simulink subsystem "PowerSplitDriveUnitBasic_refsub"  (R2020b)
settings: Solver=VariableStepAuto  StartTime=0.0  StopTime=10.0  RelTol=1e-3
libraries: nesl_utility x4, fl_lib x2
settings Model: Creator=isaacito  LastModifiedBy=isaacito

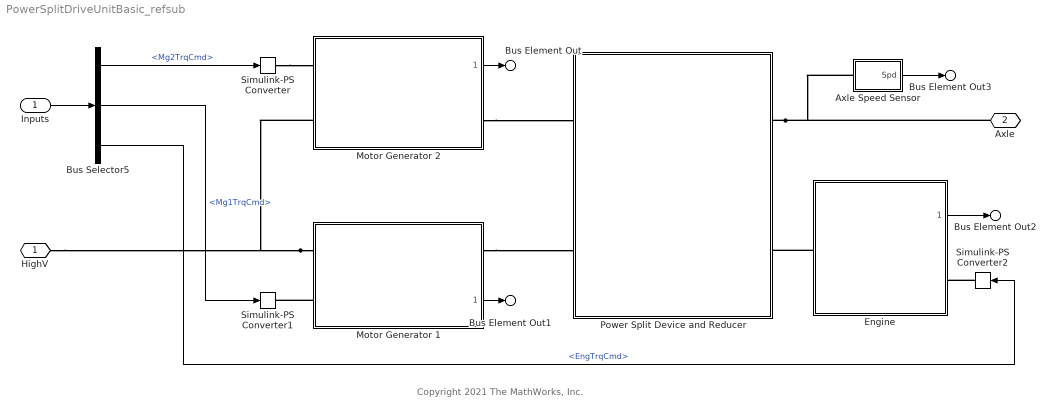
== system PowerSplitDriveUnitBasic_refsub ==
  note: Copyright 2021 The MathWorks, Inc.
  Inputs : Inport
  Axle Speed Sensor : Subsystem
  Bus Selector5 : BusSelector  OutputSignals=Mg2TrqCmd,Mg1TrqCmd,EngTrqCmd
  Engine : Subsystem  ReferencedSubsystem=EngineBasic_refsub
  Motor Generator 1 : Subsystem  ReferencedSubsystem=MotorGenerator1Basic_refsub
      settings: PortSchema="{\"entries\":[{\"content\":{\"sides\":[{\"content\":{\"connectorIds\":[\"LConn1\",\"LConn2\"]},\"type\":\"ConnectorPlacement.EquallySpacedRectSide\",\"uuid\":\"3f13e6b9-9785-470e-b4e7-2230544192d3\"},{\"content\":{\"connectorIds\":[\"RConn1\",\"Out1\"],\"side\":\"RIGHT\"},\"type\":\"ConnectorPlacement.EquallySpacedRectSide\",\"uuid\":\"c86dc6d1-f3ea-46c4-b113-258136dcfee4\"},{\"content\":{\"connectorIds\":[],\"side\":\"TOP\"},\"type\":\"ConnectorPlacement.EquallySpacedRectSide\",\"uuid\":\"633c827b-a9f1-4506-b379-ba2a2b41c3a4\"},{\"content\":{\"connectorIds\":[],\"side\":\"HIDDEN\"},\"type\":\"ConnectorPlacement.EquallySpacedRectSide\",\"uuid\":\"493696b9-c4b5-4599-b165-b63d9ea3db6c\"}]},\"type\":\"ConnectorPlacement.EquallySpacedConnector\",\"uuid\":\"29b0ca39-3f61-4a79-b1ec-51b22406ccf5\"}],\"packageUris\":[\"http://schema.mathworks.com/mf0/Connector/R2020b\"],\"version\":\"1.0\"}"
  Motor Generator 2 : Subsystem  ReferencedSubsystem=MotorGenerator2Basic_refsub
      settings: PortSchema="{\"entries\":[{\"content\":{\"sides\":[{\"content\":{\"connectorIds\":[\"LConn2\",\"LConn1\"]},\"type\":\"ConnectorPlacement.EquallySpacedRectSide\",\"uuid\":\"fb1ae627-2a11-4cdc-b40f-1f1ad643affe\"},{\"content\":{\"connectorIds\":[\"Out1\",\"RConn1\"],\"side\":\"RIGHT\"},\"type\":\"ConnectorPlacement.EquallySpacedRectSide\",\"uuid\":\"00f90b97-65a5-4f07-9d46-c4d934bbcebd\"},{\"content\":{\"connectorIds\":[],\"side\":\"TOP\"},\"type\":\"ConnectorPlacement.EquallySpacedRectSide\",\"uuid\":\"1403ad56-fcb4-428e-96ec-7b36e4f507b4\"},{\"content\":{\"connectorIds\":[],\"side\":\"HIDDEN\"},\"type\":\"ConnectorPlacement.EquallySpacedRectSide\",\"uuid\":\"421b449c-9b3e-4f4b-a79f-ec7613821770\"}]},\"type\":\"ConnectorPlacement.EquallySpacedConnector\",\"uuid\":\"1887aacf-d3d5-4d1b-946b-79f82bd43283\"}],\"packageUris\":[\"http://schema.mathworks.com/mf0/Connector/R2020b\"],\"version\":\"1.0\"}"
  Power Split Device and Reducer : Subsystem  ReferencedSubsystem=PowerSplitDeviceBasic_refsub
  Simulink-PS Converter : nesl_utility/Simulink-PS Converter  PhysicalDomain=network_engine_domain  SubClassName=ps_input  LeftPortType=input  RightPortType=output  PseudoPeriodic=off  Frequencies=[]  NoiseDistribution=none  NoiseParameters=[]  Unit=N*m  AffineConversion=off  FilteringAndDerivatives=provide  SimscapeFilterOrder=1  InputFilterTimeConstant=0.001  UdotUserProvided=0
  Simulink-PS Converter1 : nesl_utility/Simulink-PS Converter  PhysicalDomain=network_engine_domain  SubClassName=ps_input  LeftPortType=input  RightPortType=output  PseudoPeriodic=off  Frequencies=[]  NoiseDistribution=none  NoiseParameters=[]  Unit=N*m  AffineConversion=off  FilteringAndDerivatives=provide  SimscapeFilterOrder=1  InputFilterTimeConstant=0.001  UdotUserProvided=0
  Simulink-PS Converter2 : nesl_utility/Simulink-PS Converter  PhysicalDomain=network_engine_domain  SubClassName=ps_input  LeftPortType=input  RightPortType=output  PseudoPeriodic=off  Frequencies=[]  NoiseDistribution=none  NoiseParameters=[]  Unit=N*m  AffineConversion=off  FilteringAndDerivatives=provide  SimscapeFilterOrder=1  InputFilterTimeConstant=0.001  UdotUserProvided=0
  HighV : PMIOPort  Side=Left
  Axle : PMIOPort  Port=2  Side=Right
  Bus Element Out : Outport  PortName=Info  Element=mg2
  Bus Element Out1 : Outport  PortName=Info  Element=mg1
  Bus Element Out2 : Outport  PortName=Info  Element=eng
  Bus Element Out3 : Outport  PortName=Info  Element=AxleSpd
  wires:
  Motor Generator 2/1 -> Bus Element Out/1
  Motor Generator 1/1 -> Bus Element Out1/1
  Engine/1 -> Bus Element Out2/1
  Bus Selector5/3 -> Simulink-PS Converter2/1  "<EngTrqCmd>"
  Bus Selector5/2 -> Simulink-PS Converter1/1  "<Mg1TrqCmd>"
  Inputs/1 -> Bus Selector5/1
  Axle Speed Sensor/1(Spd) -> Bus Element Out3/1
  Bus Selector5/1 -> Simulink-PS Converter/1  "<Mg2TrqCmd>"
  connections:
  Motor Generator 1/LConn1 -- Motor Generator 2/LConn1 -- HighV/RConn1
  Power Split Device and Reducer/RConn1 -- Axle Speed Sensor/LConn1 -- Axle/RConn1
  Engine/LConn1 -- Power Split Device and Reducer/RConn2
  Motor Generator 2/RConn1 -- Power Split Device and Reducer/LConn1
  Simulink-PS Converter2/RConn1 -- Engine/RConn1
  Motor Generator 1/RConn1 -- Power Split Device and Reducer/LConn2
  Simulink-PS Converter/RConn1 -- Motor Generator 2/LConn2
  Motor Generator 1/LConn2 -- Simulink-PS Converter1/RConn1

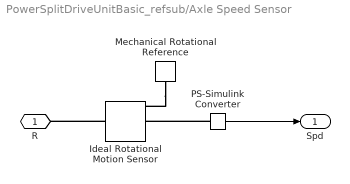
== system PowerSplitDriveUnitBasic_refsub/Axle Speed Sensor ==
  Ideal Rotational Motion Sensor : fl_lib/Mechanical/Mechanical Sensors/Ideal Rotational Motion Sensor  wrap_angle=simscape.enum.onoff.off  offset=0 rad
  Mechanical Rotational Reference : fl_lib/Mechanical/Rotational Elements/Mechanical Rotational Reference
  PS-Simulink Converter : nesl_utility/PS-Simulink Converter  PhysicalDomain=network_engine_domain  SubClassName=ps_output  LeftPortType=input  RightPortType=output  PseudoPeriodic=off  Frequencies=[]  Unit=rpm  AffineConversion=off
  R : PMIOPort  Side=Left
  Spd : Outport
  wires:
  PS-Simulink Converter/1 -> Spd/1
  connections:
  Ideal Rotational Motion Sensor/LConn1 -- R/RConn1
  PS-Simulink Converter/LConn1 -- Ideal Rotational Motion Sensor/RConn2
  Mechanical Rotational Reference/LConn1 -- Ideal Rotational Motion Sensor/RConn1
